simulink model "Tutorial3_part1"  (R2020b)
settings: Solver=FixedStepAuto  StartTime=0.0  StopTime=inf  RelTol=1e-3  EnableMultiTasking=on
libraries: simulink x1, arduinolib x1, arduinowifilib x1
settings Model: SILPILModeSetting=veronly  EnablePacing=on  ExtModeTrigDuration=2  Creator=helve  LastModifiedBy=helve
settings OptimizationCC: EnhancedBackFolding=on  PassReuseOutputArgsAs=Individual arguments  ZeroExternalMemoryAtStartup=off  ZeroInternalMemoryAtStartup=off  MaxStackSize=64  OptimizeBlockOrder=speed  DifferentSizesBufferReuse=on  OptimizationCustomize=off  EfficientTunableParamExpr=on
settings DebuggingCC: ParameterTunabilityLossMsg=error
settings HardwareCC: ProdBitPerPointer=32  ProdBitPerSizeT=32  ProdBitPerPtrDiffT=32  ProdLargestAtomicInteger=Long  ProdLargestAtomicFloat=Double  ProdWordSize=32  ProdHWDeviceType=ARM Compatible->ARM Cortex
settings SFSimCC: MATLABDynamicMemAlloc=off
settings RTWCC: Description=Embedded Coder  SystemTargetFile=ert.tlc  HardwareBoard=Arduino Nano 33 IoT  TemplateMakefile=ert_default_tmf  Toolchain=Arduino ARM  BuildConfiguration=Faster Runs
settings CodeAppCC: ForceParamTrailComments=on  IgnoreCustomStorageClasses=off  OperatorAnnotations=on  SimulinkDataObjDesc=on  SFDataObjDesc=on  InsertBlockDesc=on
settings ERTTargetCC: SupportContinuousTime=on  SupportVariableSizeSignals=on  ExtModeStaticAllocSize=8192

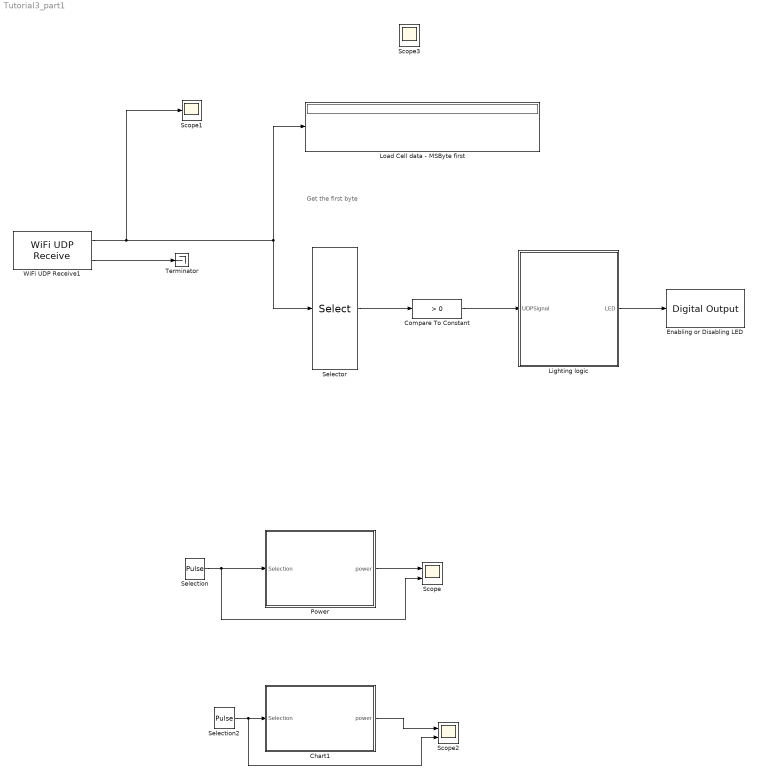
== system Tutorial3_part1 ==
  note: Get the first byte
  Chart1 : Stateflow chart  TreatAsAtomicUnit=on
  Compare To Constant : simulink/Logic and Bit Operations/Compare To Constant  relop=>  const=0  OutDataTypeStr=boolean
  Enabling or Disabling LED : arduinolib/Digital Output  pinNumber=3  Direction=output  blockPlatform=arduino
  Lighting logic : Stateflow chart  TreatAsAtomicUnit=on
  Load Cell data - MSByte first : Display
  Power : Stateflow chart  TreatAsAtomicUnit=on
  Scope : Scope  NumInputPorts=2
  Scope1 : Scope
  Scope2 : Scope  NumInputPorts=2
  Scope3 : Scope
  Selection : DiscretePulseGenerator  PulseType=Time based  Period=6  PulseWidth=10  PhaseDelay=1
  Selection2 : DiscretePulseGenerator  PulseType=Time based  Period=6  PulseWidth=10  PhaseDelay=1
  Selector : Selector  InputPortWidth=14  IndexOptions=Index vector (dialog)  Indices=[1]  OutputSizes=1
  Terminator : Terminator
  WiFi UDP Receive1 : arduinowifilib/WiFi UDP Receive  localport=50001  DataType=uint8  DataLength=14  SampleTime_=1  wifiUDPIndex=0  blockPlatform=ARDUINO  isARMArch=true
      settings: SourceProductBaseCode=ARDUINO
  wires:
  Selection/1 -> Scope/2, Power/1(Selection)
  Power/1(power) -> Scope/1
  Selection2/1 -> Chart1/1(Selection), Scope2/2
  Chart1/1(power) -> Scope2/1
  WiFi UDP Receive1/2 -> Terminator/1
  Lighting logic/1(LED) -> Enabling or Disabling LED/1
  WiFi UDP Receive1/1 -> Scope1/1, Selector/1, Load Cell data - MSByte first/1
  Selector/1 -> Compare To Constant/1
  Compare To Constant/1 -> Lighting logic/1(UDPSignal)

== stateflow chart Tutorial3_part1/Power ==
  state Init
  state Off
    en:
    power=0;
  state On
    en:
    power=1;
  (default) -> Init
  Off -> Init : {power=0}
  Init -> On : [Selection ==1 ]
  On -> Off : after(4,sec)
  data: Selection input; power output

== stateflow chart Tutorial3_part1/Chart1 ==
  state Off
    en:
    power=0;
  state On
    power=1;
  (default) -> Off
  On -> Off : after(4,sec) {power=0}
  Off -> On : [Selection ==1]
  data: power output; Selection input

== stateflow chart Tutorial3_part1/Lighting logic ==
  state LedOff
    LED=0;
  state LedOff1
    LED=1;
  (default) -> LedOff
  LedOff1 -> LedOff : after(4,sec){LED=0}
  LedOff -> LedOff1 : [UDPSignal>=1]
  data: UDPSignal input; LED output
